simulink subsystem "Piero_Beltran_23_z"  (R2023b)
settings: Solver=VariableStepAuto  StartTime=0.0  StopTime=10.0  RelTol=1e-3
settings Model: Creator=marqu  LastModifiedBy=marqu

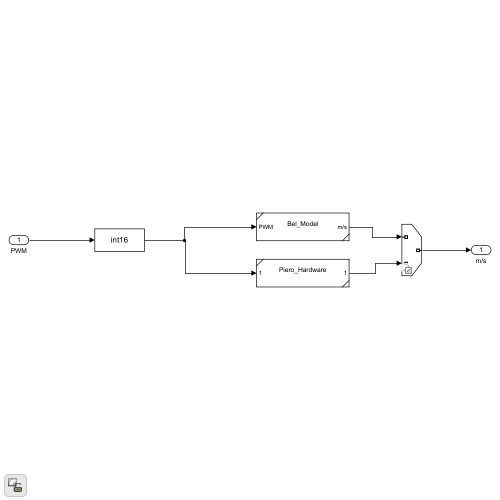
[thumbnail: Simulink's stored preview of the top-level diagram]
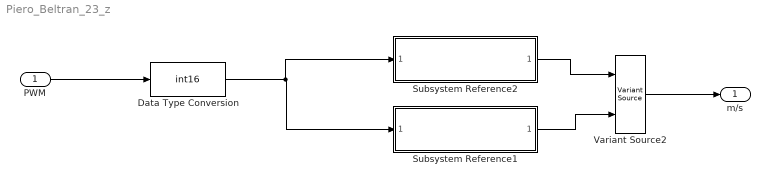
== system Piero_Beltran_23_z ==
  PWM : Inport
  Data Type Conversion : DataTypeConversion  OutDataTypeStr=int16  SaturateOnIntegerOverflow=off  RndMeth=Floor
  Subsystem Reference1 : Subsystem  ReferencedSubsystem=Piero_Hardware
  Subsystem Reference2 : Subsystem  ReferencedSubsystem=PieroBel_Model_z
  Variant Source2 : VariantSource  VariantControlMode=sim codegen switching
  m/s : Outport
  wires:
  Data Type Conversion/1 -> Subsystem Reference1/1, Subsystem Reference2/1
  PWM/1 -> Data Type Conversion/1
  Subsystem Reference2/1 -> Variant Source2/1
  Subsystem Reference1/1 -> Variant Source2/2
  Variant Source2/1 -> m/s/1
